simulink model "transmisor"  (R2020b)
settings: Solver=FixedStepDiscrete  StartTime=0.0  StopTime=1  RelTol=1e-3
values from neighbouring files (symbols this model uses):
  imagen = imread('italy.jpg')    [cargar_imagen.m]
settings Model: Creator=SALA 321  LastModifiedBy=SALA 321

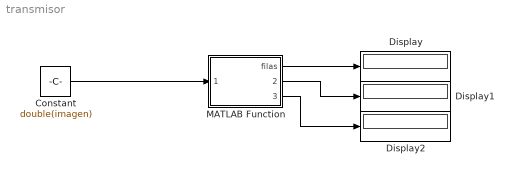
== system transmisor ==
  Constant : Constant  Value=double(imagen)  VectorParams1D=off
  Display : Display
  Display1 : Display
  Display2 : Display
  MATLAB Function : MATLAB Function  TreatAsAtomicUnit=on
  wires:
  Constant/1 -> MATLAB Function/1(imagen)
  MATLAB Function/1(filas) -> Display/1
  MATLAB Function/2(columnas) -> Display1/1
  MATLAB Function/3(canales) -> Display2/1

== matlab function transmisor/MATLAB Function ==
  data: imagen input; filas output; columnas output; canales output
function [filas, columnas, canales] = verificar_imagen(imagen)
    [filas, columnas, canales] = size(imagen);
end
